simulink model "d_7_11_8"  (R2025a)
settings: Solver=VariableStepAuto  StartTime=0.0  StopTime=100  RelTol=1e-3
settings Model: Creator=Korisnik  LastModifiedBy=Korisnik

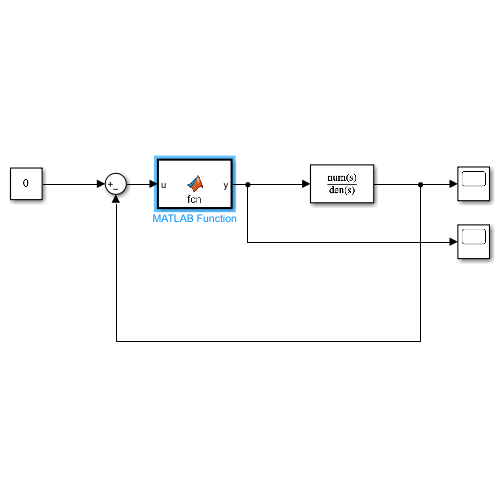
[thumbnail: Simulink's stored preview of the top-level diagram]
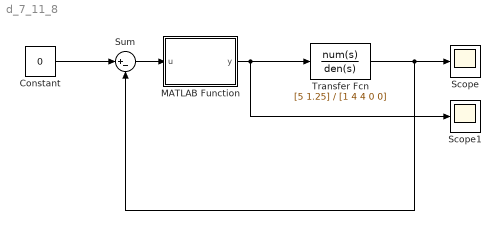
== system d_7_11_8 ==
  Constant : Constant  Value=0
  MATLAB Function : MATLAB Function  TreatAsAtomicUnit=on
  Scope : Scope
      settings: ActiveDisplayYMinimum=-0.73697413400932754  ActiveDisplayYMaximum=0.31886120611056612
  Scope1 : Scope
      settings: ActiveDisplayYMinimum=-0.73697413400932754  ActiveDisplayYMaximum=0.31886120611056612
  Sum : Sum  Inputs=|+-
  Transfer Fcn : TransferFcn  Numerator=[5 1.25]  Denominator=[1 4 4 0 0]
  wires:
  Transfer Fcn/1 -> Sum/2, Scope/1
  Constant/1 -> Sum/1
  Sum/1 -> MATLAB Function/1(u)
  MATLAB Function/1(y) -> Scope1/1, Transfer Fcn/1

== matlab function d_7_11_8/MATLAB Function ==
  data: u input; y output
function y = fcn(u)
A = 1;
B = 1.5;
if u >= B
    y = 1;
elseif u > A
    y = - 2 + 2*u;
elseif u > -A
    y = 0
elseif u > -B
    y = 2 + 2*u;
else
    y = -1
end
end
